simulink model "Motor_controller"  (R2021b)
settings: Solver=VariableStepAuto  StartTime=0.0  StopTime=10.0  RelTol=1e-3
libraries: instrumentseriallib x4
settings Model: Creator=ASUS  LastModifiedBy=ASUS

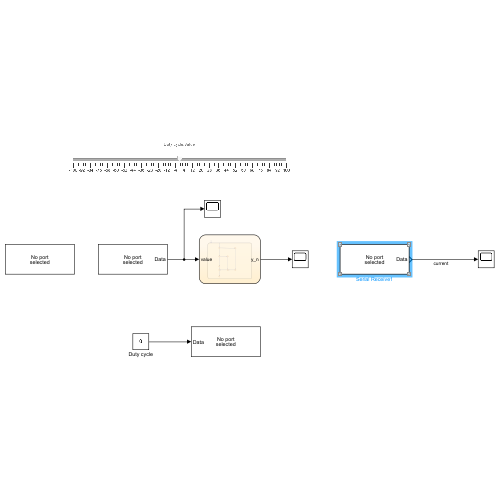
[thumbnail: Simulink's stored preview of the top-level diagram]
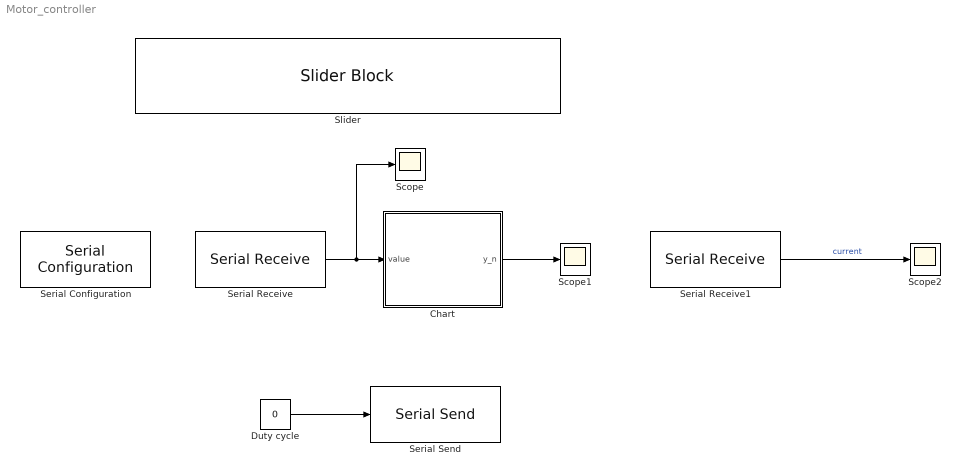
== system Motor_controller ==
  Chart : Stateflow chart  TreatAsAtomicUnit=on
  Duty cycle : Constant  Value=0
  Scope : Scope
  Scope1 : Scope
  Scope2 : Scope
  Serial Configuration : instrumentseriallib/Serial Configuration  Priority=-200000  Port=<Select a port...>  ComPort=<Select a port...>  BaudRate=1152000  DataBits=8  Parity=none  StopBits=1  ByteOrder=little-endian  FlowControl=none  Timeout=10  SimulateUsing=Interpreted execution  BlockInModel=on
  Serial Receive : instrumentseriallib/Serial Receive  Priority=1  Port=<Select a port...>  ComPort=<Select a port...>  DataType=uint16  SaveDataType=uint8  ToggleHeader=on  Header=[73 109 64 99]  ToggleTerminator=on  Terminator=Custom terminator  CustomTerminator=[126]  ToggleDataSize=on  DataSize=[1 1]  EnableBlockingMode=on  ActionDataUnavailable=Output last received value  ActionWhenDataUnavailable=Output last received value  CustomValue=0  SampleTime=0.01  SimulateUsing=Interpreted execution  BlockInModel=on
  Serial Receive1 : instrumentseriallib/Serial Receive  Priority=1  Port=<Select a port...>  ComPort=<Select a port...>  DataType=uint16  SaveDataType=uint8  ToggleHeader=on  Header=[73 109 64 100]  ToggleTerminator=on  Terminator=Custom terminator  CustomTerminator=[126]  ToggleDataSize=on  DataSize=[1 1]  EnableBlockingMode=on  ActionDataUnavailable=Output last received value  ActionWhenDataUnavailable=Output last received value  CustomValue=0  SampleTime=0.01  SimulateUsing=Interpreted execution  BlockInModel=on
  Serial Send : instrumentseriallib/Serial Send  Priority=1  Port=<Select a port...>  ComPort=<Select a port...>  Header=[73 109 64 99]  Terminator=Custom terminator  CustomTerminator=[126]  EnableBlockingMode=on  SimulateUsing=Interpreted execution  BlockInModel=on
  Slider : SliderBlock  ScaleMin=-100
  wires:
  Serial Receive/1 -> Chart/1(value), Scope/1
  Chart/1(y_n) -> Scope1/1
  Duty cycle/1 -> Serial Send/1
  Serial Receive1/1 -> Scope2/1  "current"

== stateflow chart Motor_controller/Chart ==
  state Unwrap
    Unwrap -> (junction 56)
    (junction 56) -> (junction 64) [order 1] : [value-last_value>=1500]
    (junction 56) -> (junction 59) [order 2]
    (junction 64) -> (junction 71) : {step = step-3071;}
    (junction 59) -> (junction 69) [order 1] : [value-last_value<=-1500]
    (junction 59) -> (junction 60) [order 2]
    (junction 69) -> (junction 70) : {step = step+3071;}
    (junction 60) -> (junction 103)
    (junction 70) -> (junction 103)
    (junction 71) -> (junction 70)
    (junction 103) -> (junction 104) : {y_n = value+step;
        |     last_value = value;}
  (default) -> Unwrap
  data: step local; last_value local; y_n output; value input
